simulink model "ADP_1LinkRobot_PE_3Player_ModFree_Nash"  (R2018b)
settings: Solver=ode113  StartTime=0.0  StopTime=10  FixedStep=1/5000  MaxStep=0.001  RelTol=1e-3  AbsTol=1e-3  EnableMultiTasking=on
InitFcn:
  | ADP_1LinkRobot_PE_3Player_ModFree_Nash_PreSim
values from neighbouring files (symbols this model uses):
  alpha = 200    [ADP_1LinkRobot_PE_3Player_ModFree_Nash_PreSim.m]    (also in ADP_1LinkRobot_PE_ModFree_Nash_PreSim.m)
  beta1 = 0.2    [ADP_1LinkRobot_PE_3Player_ModFree_Nash_PreSim.m]    (also in ADP_1LinkRobot_PE_ModFree_Nash_PreSim.m)
  beta_1 = 0.03    [ADP_1LinkRobot_PE_3Player_ModFree_Nash_PreSim.m]    (also in ADP_1LinkRobot_PE_ModFree_Nash_PreSim.m)
  beta_2 = 0.03    [ADP_1LinkRobot_PE_3Player_ModFree_Nash_PreSim.m]    (also in ADP_1LinkRobot_PE_ModFree_Nash_PreSim.m)
  beta_3 = 0.03    [ADP_1LinkRobot_PE_3Player_ModFree_Nash_PreSim.m]
  etaa1_1 = 0.1    [ADP_1LinkRobot_PE_3Player_ModFree_Nash_PreSim.m]    (also in ADP_1LinkRobot_PE_ModFree_Nash_PreSim.m)
  etaa1_2 = 0.1    [ADP_1LinkRobot_PE_3Player_ModFree_Nash_PreSim.m]    (also in ADP_1LinkRobot_PE_ModFree_Nash_PreSim.m)
  etaa1_3 = 0.1    [ADP_1LinkRobot_PE_3Player_ModFree_Nash_PreSim.m]
  etaa2_1 = 20    [ADP_1LinkRobot_PE_3Player_ModFree_Nash_PreSim.m]    (also in ADP_1LinkRobot_PE_ModFree_Nash_PreSim.m)
  etaa2_2 = 20    [ADP_1LinkRobot_PE_3Player_ModFree_Nash_PreSim.m]    (also in ADP_1LinkRobot_PE_ModFree_Nash_PreSim.m)
  etaa2_3 = 20    [ADP_1LinkRobot_PE_3Player_ModFree_Nash_PreSim.m]
  etac1_1 = 25    [ADP_1LinkRobot_PE_3Player_ModFree_Nash_PreSim.m]    (also in ADP_1LinkRobot_PE_ModFree_Nash_PreSim.m)
  etac1_2 = 10    [ADP_1LinkRobot_PE_3Player_ModFree_Nash_PreSim.m]    (also in ADP_1LinkRobot_PE_ModFree_Nash_PreSim.m)
  etac1_3 = 10    [ADP_1LinkRobot_PE_3Player_ModFree_Nash_PreSim.m]
  gamma = 5    [ADP_1LinkRobot_PE_3Player_ModFree_Nash_PreSim.m]    (also in ADP_1LinkRobot_PE_ModFree_Nash_PreSim.m)
  Gamma0_1 = 5000*eye(L)    [ADP_1LinkRobot_PE_3Player_ModFree_Nash_PreSim.m]    (also in ADP_1LinkRobot_PE_ModFree_Nash_PreSim.m)
  Gamma0_2 = 5000*eye(L)    [ADP_1LinkRobot_PE_3Player_ModFree_Nash_PreSim.m]    (also in ADP_1LinkRobot_PE_ModFree_Nash_PreSim.m)
  Gamma0_3 = 5000*eye(L)    [ADP_1LinkRobot_PE_3Player_ModFree_Nash_PreSim.m]
  GammaDNN = 0.1    [ADP_1LinkRobot_PE_3Player_ModFree_Nash_PreSim.m]    (also in ADP_1LinkRobot_PE_ModFree_Nash_PreSim.m)
  k = 300    [ADP_1LinkRobot_PE_3Player_ModFree_Nash_PreSim.m]    (also in ADP_1LinkRobot_PE_ModFree_Nash_PreSim.m)
  nu0 = [0;0]    [ADP_1LinkRobot_PE_3Player_ModFree_Nash_PreSim.m]    (also in ADP_1LinkRobot_PE_ModFree_Nash_PreSim.m)
  pecutoff = .3    (= 0.3)    [ADP_1LinkRobot_PE_3Player_ModFree_Nash_PreSim.m]    (also in ADP_1LinkRobot_PE_ModFree_Nash_PreSim.m)
  Q_1 = 2*eye(2)    [ADP_1LinkRobot_PE_3Player_ModFree_Nash_PreSim.m]    (also in ADP_1LinkRobot_PE_ModFree_Nash_PreSim.m)
  Q_2 = eye(2)    [ADP_1LinkRobot_PE_3Player_ModFree_Nash_PreSim.m]    (also in ADP_1LinkRobot_PE_ModFree_Nash_PreSim.m)
  Q_3 = eye(2)    [ADP_1LinkRobot_PE_3Player_ModFree_Nash_PreSim.m]
  R_11 = 2    [ADP_1LinkRobot_PE_3Player_ModFree_Nash_PreSim.m]    (also in ADP_1LinkRobot_PE_ModFree_Nash_PreSim.m)
  R_12 = 2    [ADP_1LinkRobot_PE_3Player_ModFree_Nash_PreSim.m]    (also in ADP_1LinkRobot_PE_ModFree_Nash_PreSim.m)
  R_13 = 1    [ADP_1LinkRobot_PE_3Player_ModFree_Nash_PreSim.m]
  R_21 = 1    [ADP_1LinkRobot_PE_3Player_ModFree_Nash_PreSim.m]    (also in ADP_1LinkRobot_PE_ModFree_Nash_PreSim.m)
  R_22 = 1    [ADP_1LinkRobot_PE_3Player_ModFree_Nash_PreSim.m]    (also in ADP_1LinkRobot_PE_ModFree_Nash_PreSim.m)
  R_23 = 1    [ADP_1LinkRobot_PE_3Player_ModFree_Nash_PreSim.m]
  R_31 = 1    [ADP_1LinkRobot_PE_3Player_ModFree_Nash_PreSim.m]
  R_32 = 1    [ADP_1LinkRobot_PE_3Player_ModFree_Nash_PreSim.m]
  R_33 = 1    [ADP_1LinkRobot_PE_3Player_ModFree_Nash_PreSim.m]
  test = 0    [ADP_1LinkRobot_PE_3Player_ModFree_Nash_PreSim.m]    (also in ADP_1LinkRobot_PE_ModFree_Nash_PreSim.m)
  v_1 = 0.001    [ADP_1LinkRobot_PE_3Player_ModFree_Nash_PreSim.m]    (also in ADP_1LinkRobot_PE_ModFree_Nash_PreSim.m)
  v_2 = 0.001    [ADP_1LinkRobot_PE_3Player_ModFree_Nash_PreSim.m]    (also in ADP_1LinkRobot_PE_ModFree_Nash_PreSim.m)
  v_3 = 0.001    [ADP_1LinkRobot_PE_3Player_ModFree_Nash_PreSim.m]
  VfH0 = -1+2*rand(n,Lf)    [ADP_1LinkRobot_PE_3Player_ModFree_Nash_PreSim.m]    (also in ADP_1LinkRobot_PE_ModFree_Nash_PreSim.m)
  WaH0_1 = 1*WcH0_1    [ADP_1LinkRobot_PE_3Player_ModFree_Nash_PreSim.m]    (also in ADP_1LinkRobot_PE_ModFree_Nash_PreSim.m)
  WaH0_2 = 1*WcH0_2    [ADP_1LinkRobot_PE_3Player_ModFree_Nash_PreSim.m]    (also in ADP_1LinkRobot_PE_ModFree_Nash_PreSim.m)
  WaH0_3 = 1*WcH0_3    [ADP_1LinkRobot_PE_3Player_ModFree_Nash_PreSim.m]
  WcH0_1 = 1*[1 1 1]'    [ADP_1LinkRobot_PE_3Player_ModFree_Nash_PreSim.m]    (also in ADP_1LinkRobot_PE_ModFree_Nash_PreSim.m = 3*[1 1 1]')
  WcH0_2 = 1*[1 1 1]'    [ADP_1LinkRobot_PE_3Player_ModFree_Nash_PreSim.m]    (also in ADP_1LinkRobot_PE_ModFree_Nash_PreSim.m = 3*[1 1 1]')
  WcH0_3 = 1*[1 1 1]'    [ADP_1LinkRobot_PE_3Player_ModFree_Nash_PreSim.m]
  WfH0 = -1+2*rand((Lf+1),n)    [ADP_1LinkRobot_PE_3Player_ModFree_Nash_PreSim.m]    (also in ADP_1LinkRobot_PE_ModFree_Nash_PreSim.m)
  x0 = [3;-1]    [ADP_1LinkRobot_PE_3Player_ModFree_Nash_PreSim.m]    (also in ADP_1LinkRobot_PE_ModFree_Nash_PreSim.m)
  xH0 = [0;0]    [ADP_1LinkRobot_PE_3Player_ModFree_Nash_PreSim.m]    (also in ADP_1LinkRobot_PE_ModFree_Nash_PreSim.m)
settings Model: Creator=rkamalapurkar  LastModifiedBy=rushik
settings SolverCC: AutoScaleAbsTol=off
settings DataIOCC: MaxDataPoints=10000  SaveFormat=Array  SignalLoggingSaveFormat=ModelDataLogs
settings OptimizationCC: ExpressionDepthLimit=2147483647  LifeSpan=inf
settings DebuggingCC: UnderspecifiedInitializationDetection=Classic  MergeDetectMultiDrivingBlocksExec=none  SolverPrmCheckMsg=warning  FcnCallInpInsideContextMsg=warning  StateNameClashWarn=warning  SFUnexpectedBacktrackingDiag=warning  SFNoUnconditionalDefaultTransitionDiag=warning  SFExecutionAtInitializationDiag=none
settings HardwareCC: ProdBitPerPointer=32  ProdBitPerSizeT=32  ProdBitPerPtrDiffT=32  ProdLargestAtomicFloat=None  ProdIntDivRoundTo=Undefined  ProdEndianess=Unspecified  ProdWordSize=32  ProdHWDeviceType=32-bit Generic
settings ModelReferenceCC: PropagateSignalLabelsOutOfModel=off
settings SFSimCC: SimUseLocalCustomCode=off  SimParseCustomCode=off
settings RTWCC: RTWUseLocalCustomCode=off
settings CodeAppCC: StateflowObjectComments=on
settings GRTTargetCC: TargetLangStandard=C89/C90 (ANSI)  GeneratePreprocessorConditionals=Disable all  CombineOutputUpdateFcns=off  GRTInterface=on
settings ConfigComp: CovMetricSettings=dw  CovHtmlReporting=on  CovSaveCumulativeToWorkspaceVar=on  CovSaveSingleToWorkspaceVar=on  CovExternalEMLEnable=off

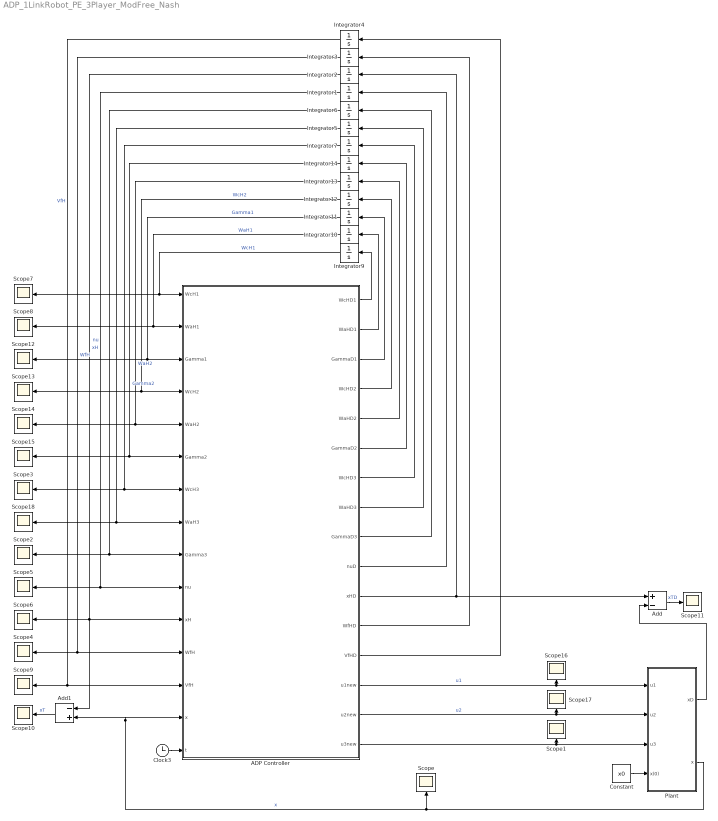
== system ADP_1LinkRobot_PE_3Player_ModFree_Nash ==
  ADP Controller : MATLAB Function  TreatAsAtomicUnit=on
  Add : Sum  Inputs=+-
  Add1 : Sum  Inputs=-+
  Clock3 : Clock
  Constant : Constant  Value=x0
  Integrator1 : Integrator  InitialCondition=nu0
  Integrator10 : Integrator  InitialCondition=WaH0_1
  Integrator11 : Integrator  InitialCondition=Gamma0_1
  Integrator12 : Integrator  InitialCondition=WcH0_2
  Integrator13 : Integrator  InitialCondition=WaH0_2
  Integrator14 : Integrator  InitialCondition=Gamma0_2
  Integrator2 : Integrator  InitialCondition=xH0
  Integrator3 : Integrator  InitialCondition=WfH0
  Integrator4 : Integrator  InitialCondition=VfH0
  Integrator5 : Integrator  InitialCondition=WaH0_3
  Integrator6 : Integrator  InitialCondition=Gamma0_3
  Integrator7 : Integrator  InitialCondition=WcH0_3
  Integrator9 : Integrator  InitialCondition=WcH0_1
  Plant : Subsystem
  Scope{,1..18} (19 alike) : Scope
  wires:
  Plant/2(x) -> Scope/1, ADP Controller/14(x), Add1/2  "x"
  Constant/1 -> Plant/4(x(0))
  ADP Controller/1(WcHD1) -> Integrator9/1
  ADP Controller/2(WaHD1) -> Integrator10/1
  ADP Controller/3(GammaD1) -> Integrator11/1
  ADP Controller/4(WcHD2) -> Integrator12/1
  ADP Controller/5(WaHD2) -> Integrator13/1
  ADP Controller/6(GammaD2) -> Integrator14/1
  ADP Controller/15(u2new) -> Plant/2(u2), Scope17/1  "u2"
  ADP Controller/14(u1new) -> Scope16/1, Plant/1(u1)  "u1"
  Clock3/1 -> ADP Controller/15(t)
  Integrator9/1 -> Scope7/1, ADP Controller/1(WcH1)  "WcH1"
  Integrator10/1 -> Scope8/1, ADP Controller/2(WaH1)  "WaH1"
  Integrator11/1 -> Scope12/1, ADP Controller/3(Gamma1)  "Gamma1"
  Integrator12/1 -> Scope13/1, ADP Controller/4(WcH2)  "WcH2"
  Integrator13/1 -> Scope14/1, ADP Controller/5(WaH2)  "WaH2"
  Integrator14/1 -> Scope15/1, ADP Controller/6(Gamma2)  "Gamma2"
  ADP Controller/10(nuD) -> Integrator1/1
  ADP Controller/11(xHD) -> Integrator2/1, Add/1
  ADP Controller/12(WfHD) -> Integrator3/1
  ADP Controller/13(VfHD) -> Integrator4/1
  Integrator1/1 -> ADP Controller/10(nu), Scope5/1  "nu"
  Integrator2/1 -> Add1/1, ADP Controller/11(xH), Scope6/1  "xH"
  Integrator3/1 -> ADP Controller/12(WfH), Scope4/1  "WfH"
  Integrator4/1 -> Scope9/1, ADP Controller/13(VfH)  "VfH"
  Plant/1(xD) -> Add/2
  Add/1 -> Scope11/1  "xTD"
  Add1/1 -> Scope10/1  "xT"
  ADP Controller/16(u3new) -> Scope1/1, Plant/3(u3)
  ADP Controller/7(WcHD3) -> Integrator7/1
  ADP Controller/8(WaHD3) -> Integrator5/1
  ADP Controller/9(GammaD3) -> Integrator6/1
  Integrator7/1 -> Scope3/1, ADP Controller/7(WcH3)
  Integrator5/1 -> Scope18/1, ADP Controller/8(WaH3)
  Integrator6/1 -> Scope2/1, ADP Controller/9(Gamma3)

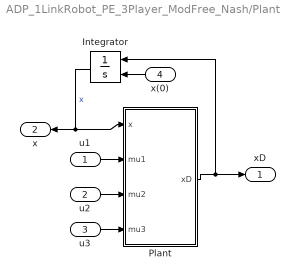
== system ADP_1LinkRobot_PE_3Player_ModFree_Nash/Plant ==
  u1 : Inport
  u2 : Inport  Port=2
  u3 : Inport  Port=3
  x(0) : Inport  Port=4
  Integrator : Integrator  InitialConditionSource=external  InitialCondition=[1;1;0.0;0.0]
  Plant : MATLAB Function  TreatAsAtomicUnit=on
  xD : Outport
  x : Outport  Port=2
  wires:
  Plant/1(xD) -> xD/1, Integrator/1
  u1/1 -> Plant/2(mu1)
  x(0)/1 -> Integrator/2
  Integrator/1 -> Plant/1(x), x/1  "x"
  u2/1 -> Plant/3(mu2)
  u3/1 -> Plant/4(mu3)

== matlab function ADP_1LinkRobot_PE_3Player_ModFree_Nash/Plant/Plant ==
  data: xD output; x input; mu1 input; mu2 input; mu3 input
function xD = dynamics(x,mu1,mu2,mu3)
%#codegen
F=[x(2)-2*x(1) ;-0.5*x(1)-x(2)+...
    0.25*x(2)*(cos(2*x(1))+2)^2+...
    0.25*x(2)*(sin(4*x(1)^2)+2)^2+...
    0.25*x(2)*(cos(4*x(1)^2)+2)^2];
G1=[0; cos(2*x(1))+2];
G2=[0; sin(4*x(1)^2)+2];
G3=[0; cos(4*x(1)^2)+2]; 
xD = F+G1*mu1+G2*mu2+G3*mu3;

== matlab function ADP_1LinkRobot_PE_3Player_ModFree_Nash/ADP Controller ==
  data: WcH1 input; WaH1 input; Gamma1 input; WcH2 input; WaH2 input; Gamma2 input; WcH3 input; WaH3 input; Gamma3 input; nu input; xH input; WfH input; VfH input; x input; t input; tf parameter; R_11 parameter; R_22 parameter; R_33 parameter; R_21 parameter; R_12 parameter; R_31 parameter; R_13 parameter; R_23 parameter; R_32 parameter; Q_1 parameter; Q_2 parameter; Q_3 parameter; etaa1_1 parameter; etaa2_1 parameter; etaa1_2 parameter; etaa2_2 parameter; etaa1_3 parameter; etaa2_3 parameter; etac1_1 parameter; etac1_2 parameter; etac1_3 parameter; v_1 parameter; v_2 parameter; v_3 parameter; pecutoff parameter; WcHD1 output; WaHD1 output; GammaD1 output; WcHD2 output; WaHD2 output; GammaD2 output; WcHD3 output; WaHD3 output; GammaD3 output; nuD output; xHD output; WfHD output; VfHD output; beta_1 parameter; u1new output; u2new output; beta_2 parameter; beta_3 parameter; test parameter; k parameter; alpha parameter; gamma parameter; beta1 parameter; GammaDNN parameter; x0 parameter; xH0 parameter; u3new output
function [WcHD1,WaHD1,GammaD1,WcHD2,WaHD2,GammaD2,WcHD3,WaHD3,GammaD3,...
    nuD,xHD,WfHD,VfHD,u1new,u2new,u3new]=control(WcH1,WaH1,Gamma1,...
    WcH2,WaH2,Gamma2,WcH3,WaH3,Gamma3,nu,xH,WfH,VfH,x,t,tf,R_11,R_22,...
    R_33,R_21,R_12,R_31,R_13,R_23,R_32,Q_1,Q_2,Q_3,etaa1_1,etaa2_1,...
    etaa1_2,etaa2_2,etaa1_3,etaa2_3,etac1_1,etac1_2,etac1_3,v_1,v_2,v_3,...
    pecutoff,beta_1,beta_2,beta_3,test,k,alpha,gamma,beta1,GammaDNN,x0,xH0)
%#codegen

G1 = [0 ; cos(2*x(1))+2];
G2 = [0 ; sin(4*x(1)^2)+2]; 
G3 = [0 ; cos(4*x(1)^2)+2]; 
phi_p =[2*x(1) 0; x(2) x(1); 0 2*x(2)];
% F=[x(2)-2*x(1) ;-0.5*x(1)-x(2)+.25*x(2)*(cos(2*x(1))+2)^2+0.25*x(2)*(sin(4*x(1)^2)+2)^2];
u1=-0.5*(R_11\G1')*phi_p'*WaH1;
u2=-0.5*(R_22\G2')*phi_p'*WaH2;
u3=-0.5*(R_33\G3')*phi_p'*WaH3;
% pe = sin(2*pi*t) + sin(exp(1)*t) + cos(5*t)^5;
% pe = (1.2-exp(.01*t))*(cos(0.2*t)^2+(sin(2*t)^2)*cos(0.1*t)+(sin(-1.2*t)^2)*cos(0.5*t)+sin(t)^5);
pe = (sin(5*pi*t) + sin(exp(1)*t) + cos(20*t)^5)+(sin(-1.2*t)^2)*cos(0.5*t)+sin(t)^5;
% pe = (sin(4*pi*t) + sin(exp(3)*t) + cos(10*t)^5);% + (1.2-exp(.01*t))*(cos(0.2*t)^2+(sin(2*t)^2)*cos(0.1*t)+(sin(-1.2*t)^2)*cos(0.5*t)+sin(t)^5);
u1new = u1 + pe*(t<=tf*pecutoff);
u2new = u2 + pe*(t<=tf*pecutoff);
u3new = u3 + pe*(t<=tf*pecutoff);

%% System ID

xT = x-xH;      
mu = (k)*xT - (k)*(x0-xH0) + nu;
nuD = (k*alpha+gamma)*xT + beta1*sign(xT);
%NN
sigmaf = (1-exp(-(VfH'*xH)))./(1+exp(-(VfH'*xH)));
sigma_f = [1; sigmaf];
fxH =  WfH'*sigma_f;   
xHD_update = fxH + G1*u1 + G2*u2 + G3*u3 + mu;   
xHD = fxH + G1*u1new + G2*u2new + G3*u3new + mu; 
sig_p_f = diag(2*exp(-VfH'*xH)./(1+exp(-VfH'*xH)).^2);
sigmaHPf = [zeros(1,length(sig_p_f)); sig_p_f];  
WfHD = (GammaDNN*sigmaHPf*VfH'*xHD_update*xT');
VfHD = (GammaDNN*xHD_update*xT'*WfH'*sigmaHPf);

%% ADP

omega = phi_p*(xHD_update);
% player 1
Gsigma1 = phi_p*G1*(R_11\G1')*phi_p'; 
Gsigma12 = phi_p*G2*(1/R_22)*R_12*(1/R_22)*G2'*phi_p'; 
Gsigma21 = phi_p*G1*(1/R_11)*R_21*(1/R_11)*G1'*phi_p';
Gsigma13 = phi_p*G3*(1/R_33)*R_13*(1/R_33)*G3'*phi_p'; 
Gsigma31 = phi_p*G1*(1/R_11)*R_31*(1/R_11)*G1'*phi_p';
Gsigma32 = phi_p*G2*(1/R_22)*R_32*(1/R_22)*G2'*phi_p'; 
Gsigma23 = phi_p*G3*(1/R_33)*R_23*(1/R_33)*G3'*phi_p';
r1 = x'*Q_1*x + u1'*R_11*u1 + u2'*R_12*u2 + u3'*R_13*u3; 
delta1 = WcH1'*omega + r1;
r2 = x'*Q_2*x + u1'*R_21*u1 + u2'*R_22*u2 + u3'*R_23*u3; 
delta2 = WcH2'*omega + r2;
r3 = x'*Q_3*x + u1'*R_31*u1 + u2'*R_32*u2 + u3'*R_33*u3; 
delta3 = WcH3'*omega + r3;
rho1 = (1+v_1*omega'*(Gamma1)*omega);
rho2 = (1+v_2*omega'*(Gamma2)*omega);
rho3 = (1+v_3*omega'*(Gamma3)*omega);
WcHD1 = (-etac1_1*Gamma1*omega*delta1/rho1)*(test==0);
GammaD1 = etac1_1*(beta_1*Gamma1-Gamma1*(omega*omega'/rho1^2)*Gamma1)*(test==0);
WaHD1 = (etaa1_1*((WcH1'-WaH1')*Gsigma1*delta1+...
    (WcH2'*Gsigma1-WaH1'*Gsigma21)*delta2+...
    (WcH3'*Gsigma1-WaH1'*Gsigma31)*delta3)'+...
    etaa2_1*(WcH1-WaH1))*(test==0);
% player 2
Gsigma2 = phi_p*G2*(R_22\G2')*phi_p'; 
WcHD2 = (-etac1_2*Gamma2*omega*delta2/rho2)*(test==0);
GammaD2 = (beta_2*Gamma2-etac1_2*Gamma2*(omega*omega'/rho2^2)*Gamma2)*(test==0);
WaHD2 = (etaa1_2*((WcH2'-WaH2')*Gsigma2*delta2+...
    (WcH1'*Gsigma2-WaH2'*Gsigma12)*delta1+...
    (WcH3'*Gsigma2-WaH2'*Gsigma32)*delta3)'+...
    etaa2_2*(WcH2-WaH2))*(test==0);
% player 3
Gsigma3 = phi_p*G3*(R_33\G3')*phi_p'; 
WcHD3 = (-etac1_3*Gamma3*omega*delta3/rho3)*(test==0);
GammaD3 = (beta_3*Gamma3-etac1_3*Gamma3*(omega*omega'/rho3^2)*Gamma3)*(test==0);
WaHD3 = (etaa1_3*((WcH3'-WaH3')*Gsigma3*delta3+...
    (WcH1'*Gsigma3-WaH3'*Gsigma13)*delta1+...
    (WcH2'*Gsigma3-WaH3'*Gsigma23)*delta2)'+...
    etaa2_3*(WcH3-WaH3))*(test==0);

%% Plant

% xD = F+G1*u1+G2*u2;
end
